simulink model "Int_control_ex_CL"  (R2018a)
settings: Solver=VariableStepAuto  StartTime=0.0  StopTime=10.0  RelTol=1e-3
undefined symbols (not defined in the file): A, B, C, D, K, simSwitch
settings Model: Creator=pala  LastModifiedBy=pala
settings DataIOCC: FinalStateName=xF_CL  SaveFinalState=on  SaveFormat=StructureWithTime  SaveState=on  SignalLogging=off  DSMLogging=off  StateSaveName=x_CL  TimeSaveName=t_CL  OutputSaveName=y_CL

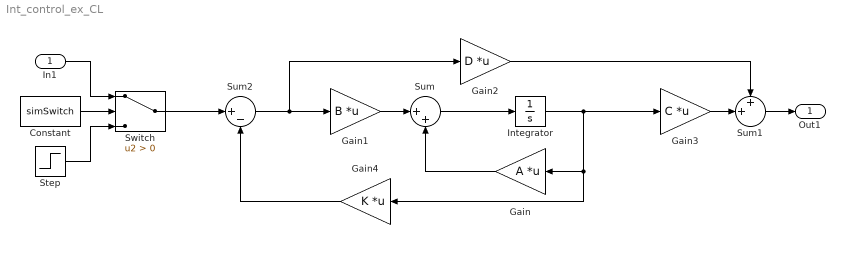
== system Int_control_ex_CL ==
  In1 : Inport
  Constant : Constant  Value=simSwitch
  Gain : Gain  Gain=A  Multiplication=Matrix(K*u)
  Gain1 : Gain  Gain=B  Multiplication=Matrix(K*u)
  Gain2 : Gain  Gain=D  Multiplication=Matrix(K*u)
  Gain3 : Gain  Gain=C  Multiplication=Matrix(K*u)
  Gain4 : Gain  Gain=K  Multiplication=Matrix(K*u)
  Integrator : Integrator
  Step : Step  SampleTime=0
  Sum : Sum  Inputs=|++
  Sum1 : Sum  Inputs=++|
  Sum2 : Sum  Inputs=|+-
  Switch : Switch  Criteria=u2 > Threshold
  Out1 : Outport
  wires:
  Gain1/1 -> Sum/1
  Gain2/1 -> Sum1/1
  Integrator/1 -> Gain3/1, Gain4/1, Gain/1
  Sum1/1 -> Out1/1
  Sum/1 -> Integrator/1
  Step/1 -> Switch/3
  Constant/1 -> Switch/2
  Gain/1 -> Sum/2
  Gain3/1 -> Sum1/2
  In1/1 -> Switch/1
  Sum2/1 -> Gain2/1, Gain1/1
  Gain4/1 -> Sum2/2
  Switch/1 -> Sum2/1
